simulink model "carAccelrator"  (R2023a)
settings: Solver=FixedStepAuto  StartTime=0.0  StopTime=4  FixedStep=0.25  MaxStep=1e-6  RelTol=1e-3
libraries: simulink x3
settings Model: Creator=gaming3  LastModifiedBy=gaming3

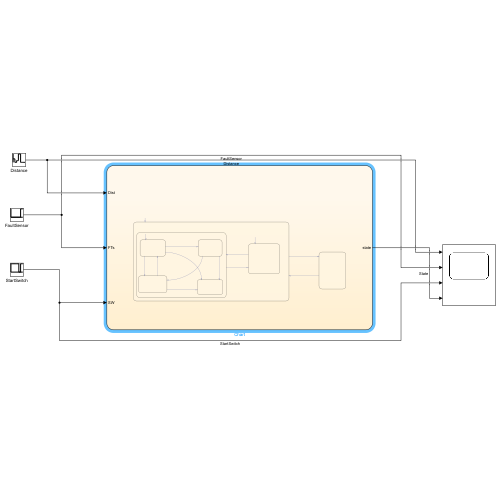
[thumbnail: Simulink's stored preview of the top-level diagram]
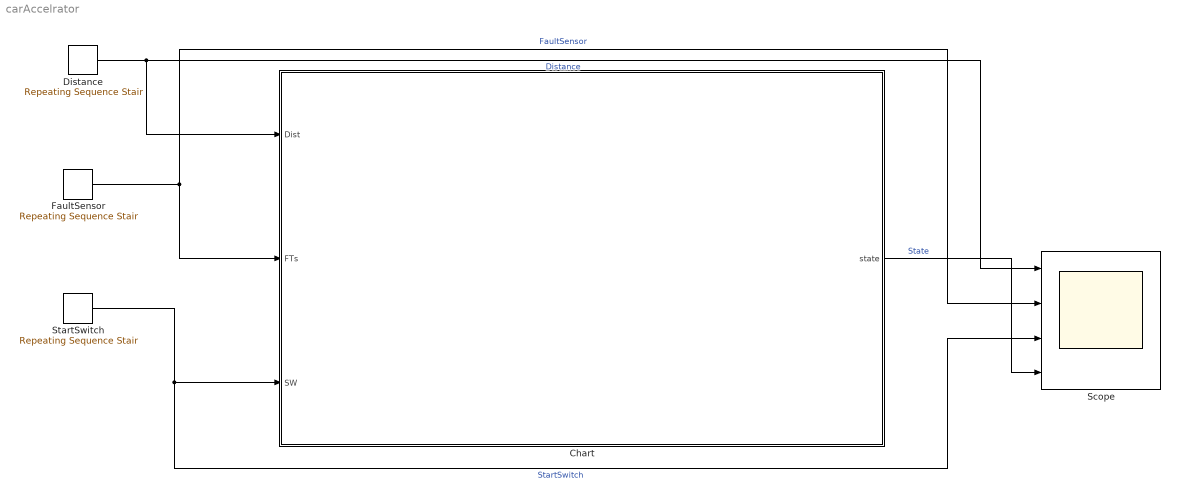
== system carAccelrator ==
  Chart : Stateflow chart  TreatAsAtomicUnit=on
  Distance : simulink/Sources/Repeating Sequence Stair  OutValues="[6 6 4 4 5 5 9 9 4 4 4 4 4  ].'"  tsamp=-1  OutMin=[]  OutMax=[]  OutDataTypeStr=double  OutputDataTypeScalingMode=double  OutDataType=fixdt(0,8)  ConRadixGroup=Best Precision: Vector-wise  OutScaling=2^-12
  FaultSensor : simulink/Sources/Repeating Sequence Stair  OutValues=[0 0 0 0 0 0 0 0 0 0 0 0 1 1 1].'  tsamp=-1  OutMin=[]  OutMax=[]  OutDataTypeStr=double  OutputDataTypeScalingMode=double  OutDataType=fixdt(0,8)  ConRadixGroup=Best Precision: Vector-wise  OutScaling=2^-12
  Scope : Scope  NumInputPorts=4
  StartSwitch : simulink/Sources/Repeating Sequence Stair  OutValues=[1 1 1 1 1 1 1 1 1 1 0 0 1 1 1].'  tsamp=-1  OutMin=[]  OutMax=[]  OutDataTypeStr=double  OutputDataTypeScalingMode=double  OutDataType=fixdt(0,8)  ConRadixGroup=Best Precision: Vector-wise  OutScaling=2^-12
  wires:
  FaultSensor/1 -> Scope/2, Chart/2(FTs)  "FaultSensor"
  StartSwitch/1 -> Scope/3, Chart/3(SW)  "StartSwitch"
  Chart/1(state) -> Scope/4  "State"
  Distance/1 -> Scope/1, Chart/1(Dist)  "Distance"

== stateflow chart carAccelrator/Chart ==
  note: state 1 = Acc
      | State -1 = braking
      | state 0=  doing nothing
      | state -2 = car stopped
      | state -3 = there is fault in system
  state Regular_system
    state ON_State
      state Braking
        en:
        state=-1;
      state Accelerating
        en:
        state = 1;
      state Nothing
        en :
        state = 0;
      state Stopping
        en :
        state = -2;
      (default) -> Accelerating
      Accelerating -> Braking [order 1] : [Dist<5]
      Accelerating -> Stopping [order 3] : [Dist<2]
      Accelerating -> Nothing [order 2] : [Dist==5]
      Nothing -> Accelerating [order 1] : [Dist>8]
      Braking -> Nothing [order 1] : [Dist==5]
      Braking -> Stopping [order 2] : [Dist<2]
      Nothing -> Stopping [order 2] : [Dist<2]
    state OFF_state
      en:
      state=-2;
    (default) -> OFF_state
    OFF_state -> ON_State : [SW==1]
    ON_State -> OFF_state : [SW==0]
  state FaultDetector
    en:
    state=-3;
  (default) -> Regular_system
  Regular_system -> FaultDetector : [FTs==1]
  FaultDetector -> Regular_system : [FTs==0]
  data: Dist input; FTs input; state output; SW input
